simulink model "velocity_plausibility"  (R2024b)
settings: Solver=FixedStepAuto  StartTime=0.0  StopTime=20  RelTol=1e-3
settings Model: Creator=aayan  LastModifiedBy=aayan
settings ConfigComp: CovEnable=on  RecordCoverage=on  CovMetricSettings=dcmwe  CovModelRefEnable=on

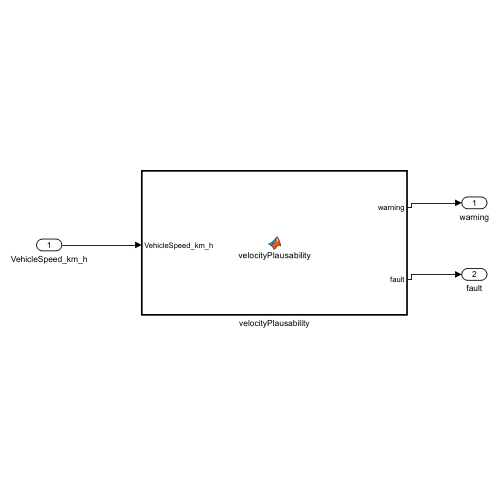
[thumbnail: Simulink's stored preview of the top-level diagram]
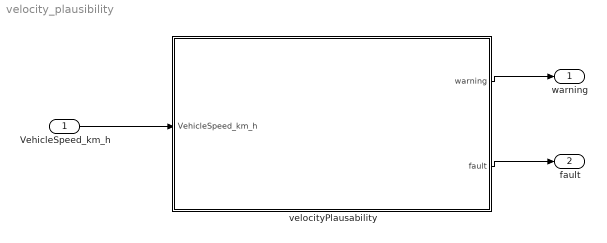
== system velocity_plausibility ==
  VehicleSpeed_km_h : Inport  OutDataTypeStr=single
  velocityPlausability : MATLAB Function  TreatAsAtomicUnit=on
  warning : Outport
  fault : Outport  Port=2
  wires:
  velocityPlausability/1(warning) -> warning/1
  velocityPlausability/2(fault) -> fault/1
  VehicleSpeed_km_h/1 -> velocityPlausability/1(VehicleSpeed_km_h)

== matlab function velocity_plausibility/velocityPlausability ==
  data: VehicleSpeed_km_h input; warning output; fault output
function [warning, fault] = velocityPlausability(VehicleSpeed_km_h)
% initialization
warning = boolean(0);
fault = boolean(0);

if (VehicleSpeed_km_h > 240|| VehicleSpeed_km_h < -60 )
    warning = boolean(1);
    fault = boolean(1);
end
